simulink model "IfElseLogic"  (R2023a)
settings: Solver=VariableStepAuto  StartTime=0.0  StopTime=10.0  RelTol=1e-3
settings Model: Creator=ADMIN  LastModifiedBy=ADMIN

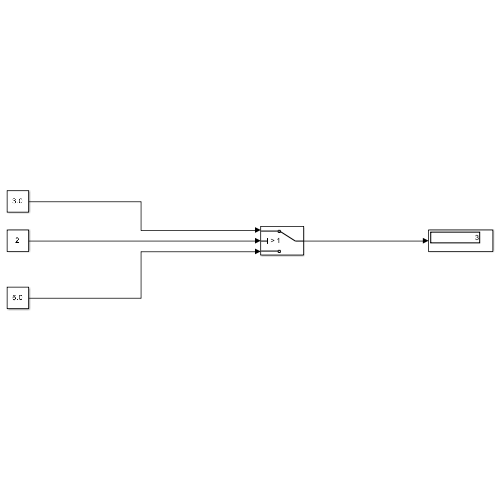
[thumbnail: Simulink's stored preview of the top-level diagram]
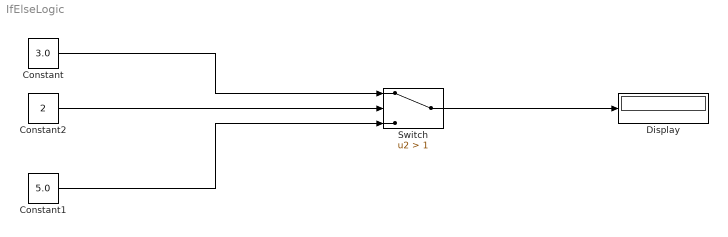
== system IfElseLogic ==
  Constant : Constant  Value=3.0
  Constant1 : Constant  Value=5.0
  Constant2 : Constant  Value=2
  Display : Display
  Switch : Switch  Criteria=u2 > Threshold  Threshold=1  SaturateOnIntegerOverflow=off  InputSameDT=off
  wires:
  Switch/1 -> Display/1
  Constant/1 -> Switch/1
  Constant2/1 -> Switch/2
  Constant1/1 -> Switch/3
